simulink model "DT_UDE_Reference"  (R2020a)
settings: Solver=FixedStepAuto  StartTime=0.0  StopTime=tstop  FixedStep=tstep  RelTol=1e-3
values from neighbouring files (symbols this model uses):
  B_n = [0;1.8]    [data.m]
  tstep = 0.01    [data.m]
  xic = [-2 1]    [data.m]
  xmic = [1 1]    [data.m]
settings Model: Creator=Maithili Shetty  LastModifiedBy=Ram Padmanabhan
settings DataIOCC: SaveOutput=off  SignalLogging=off  DSMLogging=off  SaveTime=off  ReturnWorkspaceOutputs=off

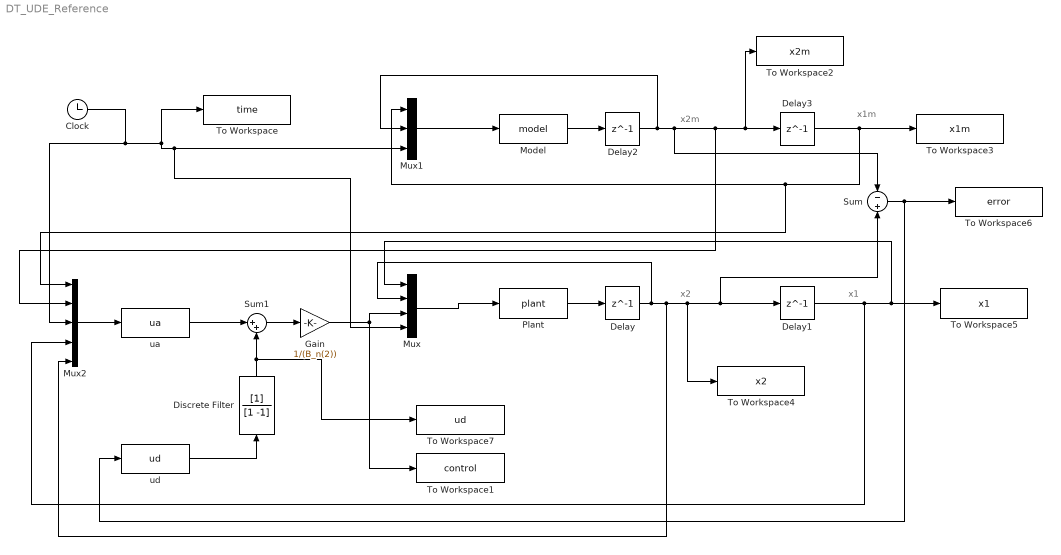
== system DT_UDE_Reference ==
  note: x1
  note: x2
  note: x2m
  note: x1m
  Clock : Clock
  Delay : Delay  DelayLength=1  InitialCondition=xic(2)  SampleTime=tstep
  Delay1 : Delay  DelayLength=1  InitialCondition=xic(1)  SampleTime=tstep
  Delay2 : Delay  DelayLength=1  InitialCondition=xmic(2)  SampleTime=tstep
  Delay3 : Delay  DelayLength=1  InitialCondition=xmic(1)  SampleTime=tstep
  Discrete Filter : DiscreteFilter  Denominator=[1 -1]  SampleTime=tstep
  Gain : Gain  Gain=1/(B_n(2))
  Model : MATLABFcn  MATLABFcn=model  OutputDimensions=1
  Mux : Mux
  Mux1 : Mux  Inputs=3
  Mux2 : Mux  Inputs=5
  Plant : MATLABFcn  MATLABFcn=plant  OutputDimensions=1
  Sum : Sum  Inputs=-+
  Sum1 : Sum  Inputs=|++
  To Workspace : ToWorkspace  VariableName=time  SampleTime=-1
  To Workspace1 : ToWorkspace  VariableName=control  SampleTime=-1
  To Workspace2 : ToWorkspace  VariableName=x2m  SampleTime=-1
  To Workspace3 : ToWorkspace  VariableName=x1m  SampleTime=-1
  To Workspace4 : ToWorkspace  VariableName=x2  SampleTime=-1
  To Workspace5 : ToWorkspace  VariableName=x1  SampleTime=-1
  To Workspace6 : ToWorkspace  VariableName=error  SampleTime=-1
  To Workspace7 : ToWorkspace  VariableName=ud  SampleTime=-1
  ua : MATLABFcn  MATLABFcn=ua  OutputDimensions=1
  ud : MATLABFcn  MATLABFcn=ud  OutputDimensions=1
  wires:
  Mux/1 -> Plant/1
  Plant/1 -> Delay/1
  Delay/1 -> Mux/2, Mux2/5, To Workspace4/1, Sum/2, Delay1/1
  Mux1/1 -> Model/1
  Model/1 -> Delay2/1
  Delay2/1 -> Sum/1, To Workspace2/1, Delay3/1, Mux2/2, Mux1/2
  Mux2/1 -> ua/1
  Clock/1 -> Mux2/3, To Workspace/1, Mux/4, Mux1/3
  Sum/1 -> To Workspace6/1, ud/1
  ud/1 -> Discrete Filter/1
  ua/1 -> Sum1/1
  Discrete Filter/1 -> To Workspace7/1, Sum1/2
  Sum1/1 -> Gain/1
  Gain/1 -> To Workspace1/1, Mux/3
  Delay1/1 -> Mux2/4, Mux/1, To Workspace5/1
  Delay3/1 -> To Workspace3/1, Mux2/1, Mux1/1
